simulink library "SY202_NCS_Library"  (R2017b)
settings: Solver=VariableStepAuto  StartTime=0.0  StopTime=10.0  RelTol=1e-3
settings Model: Creator=rodrigue  LastModifiedBy=rodrigue

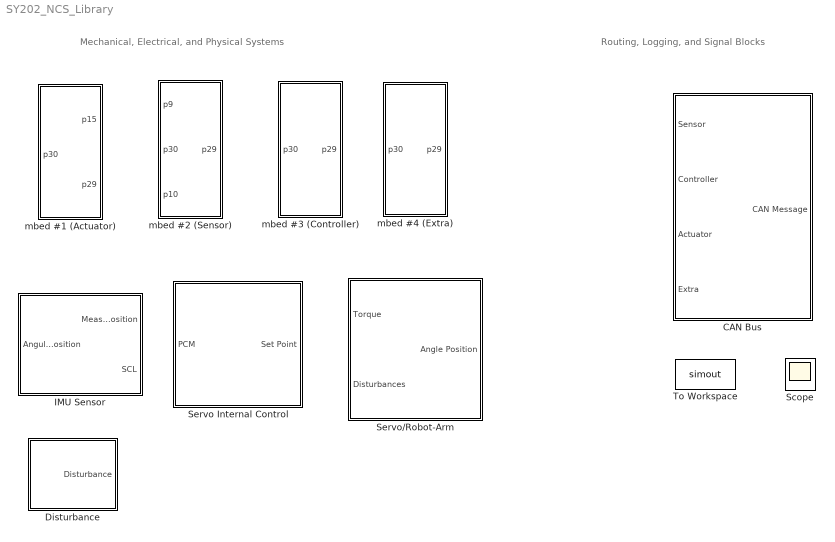
== system SY202_NCS_Library ==
  note: Mechanical, Electrical, and Physical Systems
  note: Routing, Logging, and Signal Blocks
  CAN Bus : Subsystem
      mask help: This block models a CAN Bus Network with four Nodes: a sensor, a controller, an actuator, and an extra device. The output of the CAN Bus Network is the CAN Message.
      mask Display:
      | %image('CANBUS.png')
      | color('white')
      | port_label('input',1,'{\bf{Sensor}}', 'texmode','on');
      | port_label('input',2,'{\bf{Controller}}', 'texmode','on');
      | port_label('input',3,'{\bf{Actuator}}', 'texmode','on');
      | port_label('input',4,'{\bf{Extra}}', 'texmode','on');
      | port_label('output',1,'{\bf{CAN Message}}', 'texmode','on');
  Disturbance : Subsystem  mask{DisturbanceTime=0, DisturbanceValue=0}
      mask prompts: DisturbanceTime "Start of Disturbance (s):"; DisturbanceValue "Magnitude of Disturbance (rad):"
      mask Display:
      | image('hand.jpg')
      | color('black')
      | port_label('output',1,'{\bf{Disturbance}}', 'texmode','on');
  IMU Sensor : Subsystem  AncestorBlock=SY202_NCS_Library/CAN Bus  mask{MeanSensorError=0, MeanSensorVar=0.001}
      mask prompts: MeanSensorError "Mean Error:"; MeanSensorVar "Variance:"
      mask help: This blocks model a BNO055 IMU sensor in radians. The noise (error) is assumed to have normal distribution.
      mask Display:
      | image('bno055.jpg')
      | color('white')
      | port_label('input',1,'{\bf{Angle}}', 'texmode','on');
      | port_label('output',1,'{\bf{Meas Angle - SDA}}', 'texmode','on');
      | port_label('output',2,'{\bf{Meas Angle - SCL}}', 'texmode','on');
  Scope : Scope
  Servo Internal Control : Subsystem  AncestorBlock=SY202_NCS_Library/CAN Bus  mask{MaxPW=2100, MinPW=900, MaxServo=pi/3, MinServo=-pi/3}
      mask prompts: MaxPW "Maximum PCM Value (us):"; MinPW "Minimum PCM Value (us):"; MaxServo "Maximum Angle of Servo (rad):"; MinServo "Minimum Angle of Servo (rad):"
      mask help: This block models a CAN Bus Network with four Nodes: a sensor, a controller, an actuator, and an extra device. The output of the CAN Bus Network is the CAN Message.
      mask Display:
      | image('servo.jpg')
      | color('white')
      | port_label('input',1,'{\bf{PCM/PWM}}', 'texmode','on');
      | port_label('output',1,'{\bf{Servo-Pos}}', 'texmode','on');
  Servo/Robot-Arm : Subsystem  AncestorBlock=SY202_NCS_Library/Servo Motor  mask{x0=0, xdot0=0, MaxPW=2100, MinPW=900, MaxServo=pi/3, MinServo=-pi/3}
      mask prompts: x0 "Initial Position of Arm (rad):"; xdot0 "Initial Velocity of Arm (rad/s):"; MaxPW "Maximum PCM Value (us):"; MinPW "Minimum PCM Value (us):"; MaxServo "Maximum Angle of Servo (rad):"; MinServo "Minimum Angle of Servo (rad):"
      mask help: This block models a CAN Bus Network with four Nodes: a sensor, a controller, an actuator, and an extra device. The output of the CAN Bus Network is the CAN Message.
      mask Display:
      | image('SY202Project.jpg')
      | color('black')
      | port_label('input',1,'{\bf{Servo-Pos}}', 'texmode','on');
      | port_label('input',2,'{\bf{Disturbances}}', 'texmode','on');
      | color('black')
      | port_label('output',1,'{\bf{Angle}}', 'texmode','on');
  To Workspace : ToWorkspace  VariableName=simout  SampleTime=-1
  mbed #1 (Actuator) : Subsystem  mask(Microcontroller Function){MinPW=900, MaxPW=2100}
      mask prompts: MinPW "Minimum Servo Value:"; MaxPW "Maximum Servo Value:"
      mask help:
      | This block models the implementation of the mbed microcontroller that generates the input PCW signal to the Servo Motor. It reads the controller's commands using pins p29 (CAN TD) and p30 (CAN RD) that are connected to the CAN Bus. It then sends a PCM signal to the Servo Motor using pin p15.
      |
      | Minimum and maximum servo pulse width values can be set by the user. The default values are 900 and 2100, respectively.
      mask Display:
      | image('mbed.jpeg')
      | color('orange')
      | port_label('output',1,'{\bf\fontsize{12}p15}', 'texmode','on');
      | port_label('output',2,'{\bf\fontsize{12}p29}', 'texmode','on');
      | port_label('input',1,'{\bf\fontsize{12}p30}', 'texmode','on');
      | color('white')
      | text(0.5,0.35,'\bf{mbed1}', 'texmode','on', 'horizontalAlignment', 'center')
      | %port_label('output',1,'p30')
      | %port_label('input',1,'p29')
  mbed #2 (Sensor) : Subsystem  mask(Microcontroller Function){}
      mask help: This block models the implementation of the mbed microcontroller reading the position sensor. It uses pin numbers p9 (SDA) adn P10 (SLC) to connect to read data from the sensor using the I2C communication protocol. It then sends the information to the NCS using the CAN Bus via pins p29 (CAN TD) and p30 (CAN RD).
      mask Display:
      | image('mbed.jpeg')
      | color('orange')
      | port_label('input',1,'{\bf\fontsize{12}p9 SDA}', 'texmode','on');
      | port_label('input',2,'{\bf\fontsize{12}p30}', 'texmode','on');
      | port_label('input',3,'{\bf\fontsize{12}p10 SCL}', 'texmode','on');
      | port_label('output',1,'{\bf\fontsize{12}p29}', 'texmode','on');
      | color('white')
      | text(0.5,0.35,'\bf{mbed2}', 'texmode','on', 'horizontalAlignment', 'center')
  mbed #3 (Controller) : Subsystem  mask(Microcontroller Function){DesValue=0, Kp=100, Ki=0, Offset=1400}
      mask prompts: DesValue "Desired Angular Position"; Kp "Proportional Gain (Kp)"; Ki "Integral Gain (Ki)"
      mask help:
      | This block models the implementation of a Proportional-Integral controller using the mbed microcontroller sending and receiving messages through a CAN Bus Network.  The Proportional-Integral control equation is given by:
      |
      |           PWM_Signal = -(Kp*error + Ki*integral_of_error)+Offset
      |
      | where the error is  computed as: Desired Angular Position - Measured Angular Position.
      |
      | The CAN Bus mbed pins are p29 (CAN TD) and p30 (CAN RD).
      mask Display:
      | image('mbed.jpeg')
      | color('orange')
      | port_label('output',1,'{\bf\fontsize{12}p29}', 'texmode','on');
      | port_label('input',1,'{\bf\fontsize{12}p30}', 'texmode','on');
      | color('white')
      | text(0.5,0.35,'\bf{mbed3}', 'texmode','on', 'horizontalAlignment', 'center')
  mbed #4 (Extra) : Subsystem  mask(Microcontroller Function){AttackRate=0, AttackMode=Stealth Attack, AttackMag=0, AttackTime=0}
      mask prompts: AttackRate "Rate of Attack (0 to 100%)"; AttackMode "Attack Model"; AttackMag "Attack Magnitude (rad)"; AttackTime "Start Time of Attack (s)"
      mask help:
      | This block models the implementation of an attack of deception to the CAN Bus Network. The malicious agent passes itself as the sensor and introduces false or corrupted information into the network that is later utilized by the controller to make control decisions. There are two models of attack:
      |
      | Stealth Attack:
      |
      |             False_Sensor_Data = Real_Sensor_Data + Attack_Magnitude
      |
      | Replay Attack (Variant):
      |
      |            False_Sensor_Data = Attack_Magnitude
      |
      | Rate of Attack is the attacker's rate of success at blocking and spoofing real sensor data. Choose zero for a dormant attack. Attack Bias is the malicious error introduced by the attacker. Start Time of Attack is the time at which the attacker starts injecting false data.
      |
      | The CAN Bus mbed pins used by the malicious agent are p29 (CAN TD) and p30 (CAN RD).
      mask TypeOptions AttackMode: Stealth Attack | Replay Attack (Variant)
      mask Display:
      | image('mbed.jpeg')
      | color('orange')
      | port_label('output',1,'{\bf\fontsize{12}p29}', 'texmode','on');
      | port_label('input',1,'{\bf\fontsize{12}p30}', 'texmode','on');
      | color('white')
      | text(0.5,0.35,'\bf{mbed4}', 'texmode','on', 'horizontalAlignment', 'center')

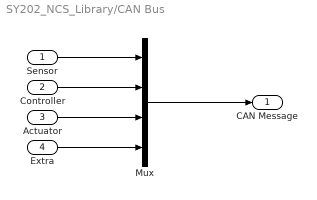
== system SY202_NCS_Library/CAN Bus ==
  Sensor : Inport
  Controller : Inport  Port=2
  Actuator : Inport  Port=3
  Extra : Inport  Port=4
  Mux : Mux
  CAN Message : Outport
  wires:
  Extra/1 -> Mux/4
  Sensor/1 -> Mux/1
  Actuator/1 -> Mux/3
  Controller/1 -> Mux/2
  Mux/1 -> CAN Message/1

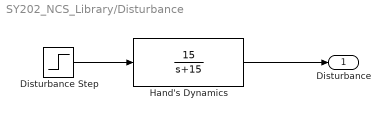
== system SY202_NCS_Library/Disturbance ==
  Disturbance Step : Step  Time=DisturbanceTime  After=DisturbanceValue  SampleTime=0
  Hand's Dynamics : TransferFcn  Numerator=[15]  Denominator=[1 15]
  Disturbance : Outport
  wires:
  Hand's Dynamics/1 -> Disturbance/1
  Disturbance Step/1 -> Hand's Dynamics/1

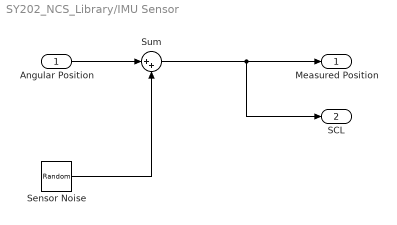
== system SY202_NCS_Library/IMU Sensor ==
  Angular Position : Inport
  Sensor Noise : RandomNumber  Mean=MeanSensorError  Variance=MeanSensorVar  SampleTime=0.1
  Sum : Sum  Inputs=|++
  Measured Position : Outport
  SCL : Outport  Port=2
  wires:
  Angular Position/1 -> Sum/1
  Sensor Noise/1 -> Sum/2
  Sum/1 -> SCL/1, Measured Position/1

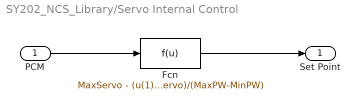
== system SY202_NCS_Library/Servo Internal Control ==
  PCM : Inport
  Fcn : Fcn  Expr=MaxServo - (u(1)-MinPW)*(MaxServo-MinServo)/(MaxPW-MinPW)
  Set Point : Outport
  wires:
  PCM/1 -> Fcn/1
  Fcn/1 -> Set Point/1

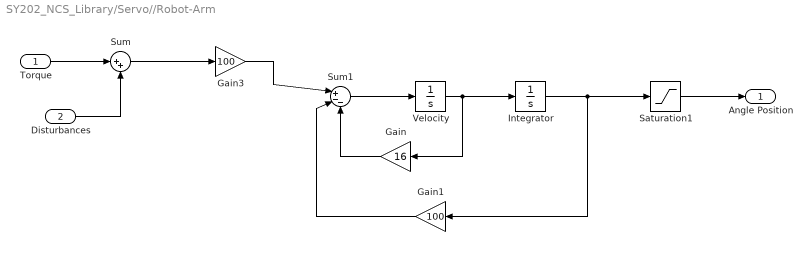
== system SY202_NCS_Library/Servo//Robot-Arm ==
  Torque : Inport
  Disturbances : Inport  Port=2
  Gain : Gain  Gain=16
  Gain1 : Gain  Gain=100
  Gain3 : Gain  Gain=100
  Integrator : Integrator  InitialCondition=x0
  Saturation1 : Saturate  UpperLimit=MaxServo  LowerLimit=MinServo
  Sum : Sum  Inputs=|++
  Sum1 : Sum  Inputs=|+--
  Velocity : Integrator  InitialCondition=xdot0
  Angle Position : Outport
  wires:
  Velocity/1 -> Gain/1, Integrator/1
  Sum1/1 -> Velocity/1
  Gain/1 -> Sum1/3
  Gain1/1 -> Sum1/2
  Gain3/1 -> Sum1/1
  Saturation1/1 -> Angle Position/1
  Disturbances/1 -> Sum/2
  Integrator/1 -> Saturation1/1, Gain1/1
  Torque/1 -> Sum/1
  Sum/1 -> Gain3/1

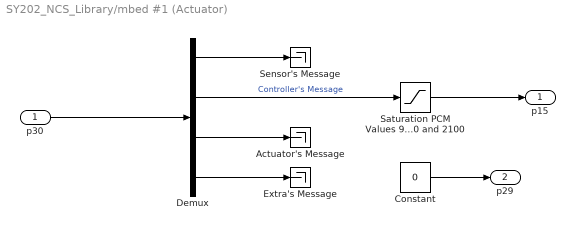
== system SY202_NCS_Library/mbed #1 (Actuator) ==
  p30 : Inport
  Actuator's Message : Terminator
  Constant : Constant  Value=0
  Demux : Demux
  Extra's Message : Terminator
  Saturation PCM Values 900 and 2100 : Saturate  UpperLimit=MaxPW  LowerLimit=MinPW
  Sensor's Message : Terminator
  p15 : Outport
  p29 : Outport  Port=2
  wires:
  p30/1 -> Demux/1
  Saturation PCM Values 900 and 2100/1 -> p15/1
  Constant/1 -> p29/1
  Demux/2 -> Saturation PCM Values 900 and 2100/1  "Controller's Message"
  Demux/3 -> Actuator's Message/1
  Demux/4 -> Extra's Message/1
  Demux/1 -> Sensor's Message/1

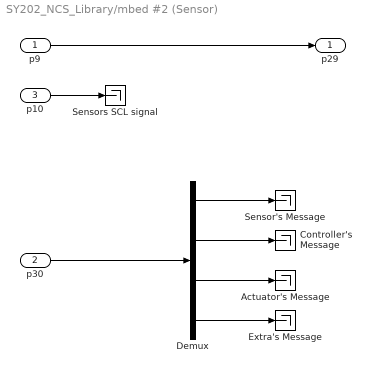
== system SY202_NCS_Library/mbed #2 (Sensor) ==
  p9 : Inport
  p30 : Inport  Port=2
  p10 : Inport  Port=3
  Actuator's Message : Terminator
  Controller's Message : Terminator
  Demux : Demux
  Extra's Message : Terminator
  Sensor's Message : Terminator
  Sensors SCL signal : Terminator
  p29 : Outport
  wires:
  p30/1 -> Demux/1
  p9/1 -> p29/1
  Demux/1 -> Sensor's Message/1
  Demux/3 -> Actuator's Message/1
  Demux/2 -> Controller's Message/1
  Demux/4 -> Extra's Message/1
  p10/1 -> Sensors SCL signal/1

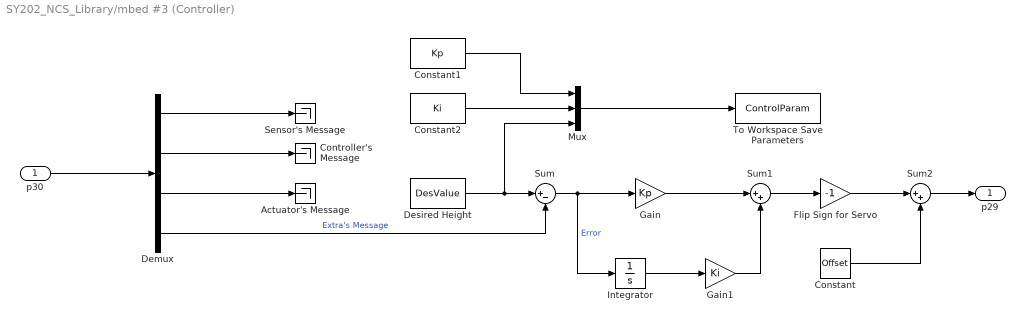
== system SY202_NCS_Library/mbed #3 (Controller) ==
  "p30 " : Inport
  Actuator's Message : Terminator
  Constant : Constant  Value=Offset
  Constant1 : Constant  Value=Kp
  Constant2 : Constant  Value=Ki
  Controller's Message : Terminator
  Demux : Demux
  Desired Height : Constant  Value=DesValue
  Flip Sign for Servo : Gain  Gain=-1
  Gain : Gain  Gain=Kp
  Gain1 : Gain  Gain=Ki
  Integrator : Integrator
  Mux : Mux  Inputs=3
  Sensor's Message : Terminator
  Sum : Sum  Inputs=|+-
  Sum1 : Sum  Inputs=|++
  Sum2 : Sum  Inputs=|++
  To Workspace Save Parameters : ToWorkspace  VariableName=ControlParam  SaveFormat=Structure  SampleTime=-1
      settings: MaxDataPoints=1
  p29 : Outport
  wires:
  Desired Height/1 -> Mux/3, Sum/1
  Sum/1 -> Integrator/1, Gain/1  "Error"
  Mux/1 -> To Workspace Save Parameters/1
  Constant1/1 -> Mux/1
  "p30 "/1 -> Demux/1
  Demux/2 -> Controller's Message/1
  Demux/3 -> Actuator's Message/1
  Demux/4 -> Sum/2  "Extra's Message"
  Demux/1 -> Sensor's Message/1
  Constant2/1 -> Mux/2
  Gain/1 -> Sum1/1
  Integrator/1 -> Gain1/1
  Gain1/1 -> Sum1/2
  Sum1/1 -> Flip Sign for Servo/1
  Sum2/1 -> p29/1
  Flip Sign for Servo/1 -> Sum2/1
  Constant/1 -> Sum2/2

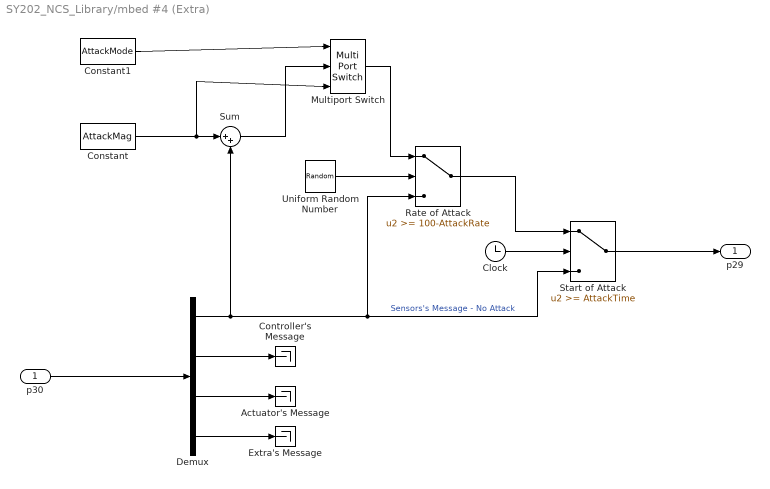
== system SY202_NCS_Library/mbed #4 (Extra) ==
  p30 : Inport
  Actuator's Message : Terminator
  Clock : Clock
  Constant : Constant  Value=AttackMag
  Constant1 : Constant  Value=AttackMode
  Controller's Message : Terminator
  Demux : Demux
  Extra's Message : Terminator
  Multiport Switch : MultiPortSwitch  Inputs=2
  Rate of Attack : Switch  Threshold=100-AttackRate
  Start of Attack : Switch  Threshold=AttackTime
  Sum : Sum  Inputs=|++
  Uniform Random Number : UniformRandomNumber  Minimum=0  Maximum=100  SampleTime=0.1
  p29 : Outport
  wires:
  p30/1 -> Demux/1
  Demux/2 -> Controller's Message/1
  Demux/3 -> Actuator's Message/1
  Demux/4 -> Extra's Message/1
  Uniform Random Number/1 -> Rate of Attack/2
  Demux/1 -> Start of Attack/3, Rate of Attack/3, Sum/2  "Sensors's Message - No Attack"
  Constant/1 -> Multiport Switch/3, Sum/1
  Clock/1 -> Start of Attack/2
  Start of Attack/1 -> p29/1
  Rate of Attack/1 -> Start of Attack/1
  Multiport Switch/1 -> Rate of Attack/1
  Constant1/1 -> Multiport Switch/1
  Sum/1 -> Multiport Switch/2
